simulink model "sim12ex7"  (Simulink 2.09)
settings: Solver=ode23  StartTime=0.0  StopTime=10  MaxStep=.050  RelTol=1e-3  AbsTol=1e-3
settings Model: SaveTime=off  SaveOutput=off  ConsistencyChecking=off  RTWTemplateMakefile=grt_vc.tmf

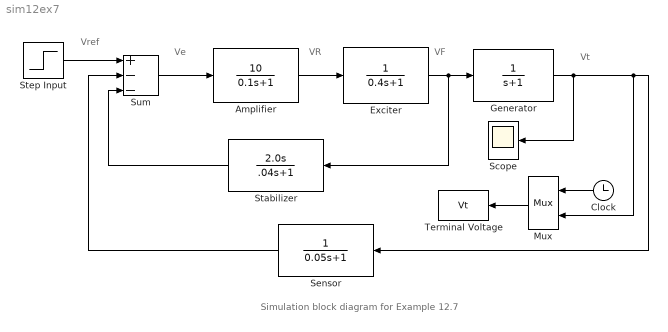
== system sim12ex7 ==
  note: Simulation block diagram for Example 12.7
  note: Vref
  note: Vt
  note: VF
  note: VR
  note: Ve
  Amplifier : TransferFcn  Numerator=[10]  Denominator="[0.1  1]"
  Clock : Clock
  Exciter : TransferFcn  Numerator=[1]  Denominator="[0.4  1]"
  Generator : TransferFcn  Numerator=[1]  Denominator="[1  1]"
  Mux : Mux  Orientation=left  Inputs=2
  Scope : Scope
      settings: TickLabels=on  TimeRange=auto  YMin=-5  YMax=5  SaveToWorkspace=off  SaveName=ScopeData
  Sensor : TransferFcn  Orientation=left  Numerator=[1]  Denominator="[0.05  1]"
  Stabilizer : TransferFcn  Orientation=left  Numerator="[ 2.0  0]"  Denominator="[.04  1]"
  Step Input : Step  Time=10  Before=1  After=1
  Sum : Sum  Inputs=+--
  Terminal Voltage : ToWorkspace  VariableName=Vt  SampleTime=0
      settings: Buffer=1000
  wires:
  Mux/1 -> Terminal Voltage/1
  Clock/1 -> Mux/1
  Generator/1 -> Mux/2, Sensor/1, Scope/1
  Exciter/1 -> Stabilizer/1, Generator/1
  Sensor/1 -> Sum/2
  Stabilizer/1 -> Sum/3
  Amplifier/1 -> Exciter/1
  Sum/1 -> Amplifier/1
  Step Input/1 -> Sum/1
